simulink model "PIDusingOPAMP"  (R2015a)
settings: Solver=ode45  StartTime=0.0  StopTime=0.008  RelTol=1e-6
libraries: fl_lib x43, nesl_utility x2, powerlib x1
settings Model: Creator=my pc  LastModifiedBy=my pc

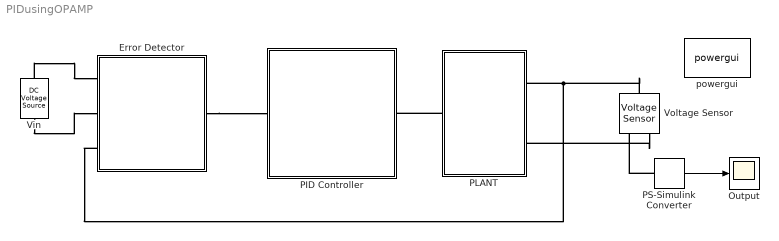
== system PIDusingOPAMP ==
  Error Detector : Subsystem
  Output : Scope
      settings: SaveName=PID
  PID Controller : Subsystem
  PLANT : Subsystem
  PS-Simulink Converter : nesl_utility/PS-Simulink Converter  PhysicalDomain=network_engine_domain  SubClassName=ps_output  LeftPortType=input  RightPortType=output  PseudoPeriodic=off  Frequencies=[]  Unit=1  AffineConversion=off
  Vin : fl_lib/Electrical/Electrical Sources/DC Voltage Source  v0=5 V
  Voltage Sensor : fl_lib/Electrical/Electrical Sensors/Voltage Sensor
  powergui : powerlib/powergui  Priority=1  SimulationMode=Continuous  SolverType=Tustin/Backward Euler (TBE)  SampleTime=50e-6  frequency=60  SPID=off  DisableSnubberDevices=off  DisableRonSwitches=off  DisableVfSwitches=off  SwTol=0  DisplayEquations=off  Interpol=off  methode=off  Ts=100  FunctionMessages=off  echomessages=off  HookPort=off  EnableUseOfTLC=off  x0status=blocks  frequencyindice=60  Pbase=100e6  ErrMax=1e-4  Iterations=50  UnitsV=kV  UnitsW=MW  buscounter=0  RestoreLinks=warning  ResistiveCurrentMeasurement=off  Frange=[0:2:500]  Ylog=off  Xlog=on  ShowGrid=off  save=off  variable=ZData  structure=0  ZoomFFT=off  StartTime=0.0  cycles=1  DisplayStyle=1  fundamental=60  FreqAxis=off  MaxFrequency=1000  frequencyindicesteady=1  RmsSteady=1  display=off
  wires:
  PS-Simulink Converter/1 -> Output/1
  connections:
  Voltage Sensor/LConn1 -- Error Detector/RConn3 -- PLANT/RConn1
  Voltage Sensor/RConn2 -- PLANT/RConn2
  Vin/LConn1 -- Error Detector/RConn1
  Vin/RConn1 -- Error Detector/RConn2
  Error Detector/LConn1 -- PID Controller/LConn1
  PS-Simulink Converter/LConn1 -- Voltage Sensor/RConn1
  PLANT/LConn1 -- PID Controller/RConn1

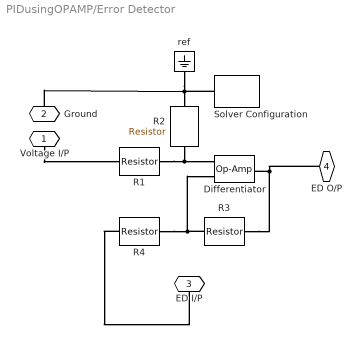
== system PIDusingOPAMP/Error Detector ==
  Differentiator : fl_lib/Electrical/Electrical Elements/Op-Amp  outI_specify=off  outI_priority=High  outI=0 A
  R{1..4} (4 alike) : fl_lib/Electrical/Electrical Elements/Resistor  R=4.7 kOhm  i_specify=off  i_priority=High  i=0 A  v_specify=off  v_priority=High  v=0 V
  Solver Configuration : nesl_utility/Solver Configuration  PhysicalDomain=network_engine_domain  SubClassName=solver  LeftPortType=input  RightPortType=generic  Accelerate=off  Tones=[]  Harmonics=[]  SimulateNoise=off  Profile=off  UseLocalSampling=off  EnableSwitchedLinearOptims=on  FrequencyDomain=off  UseCCode=off  RelTol=0.001  AbsTol=1e-06  MinStep=1e-09  ToWorkspace=off  RevertToSquareIcSolve=off  NumHomotopyIterations=100  DoDC=off  ResidualTolerance=1e-09  UseLocalSolver=off  LocalSolverChoice=NE_BACKWARD_EULER_ADVANCER  LocalSolverSampleTime=0.001  DoFixedCost=off  MaxNonlinIter=3  MaxModeIter=2  LinearAlgebra=Sparse  DelaysMemoryBudget=1024  AutomaticFiltering=on  FilteringTimeConstant=0.001
  ref : fl_lib/Electrical/Electrical Elements/Electrical Reference
  Voltage I/P : PMIOPort  Port=1  Side=Right
  Ground : PMIOPort  Port=2  Side=Right
  ED I/P : PMIOPort  Port=3  Side=Right
  ED O/P : PMIOPort  Port=4  Side=Left
  connections:
  R4/LConn1 -- ED I/P/RConn1
  Voltage I/P/RConn1 -- R1/LConn1
  R1/RConn1 -- R2/LConn1 -- Differentiator/LConn1
  ref/LConn1 -- Ground/RConn1 -- Solver Configuration/RConn1 -- R2/RConn1
  R4/RConn1 -- R3/RConn1 -- Differentiator/LConn2
  R3/LConn1 -- ED O/P/RConn1 -- Differentiator/RConn1

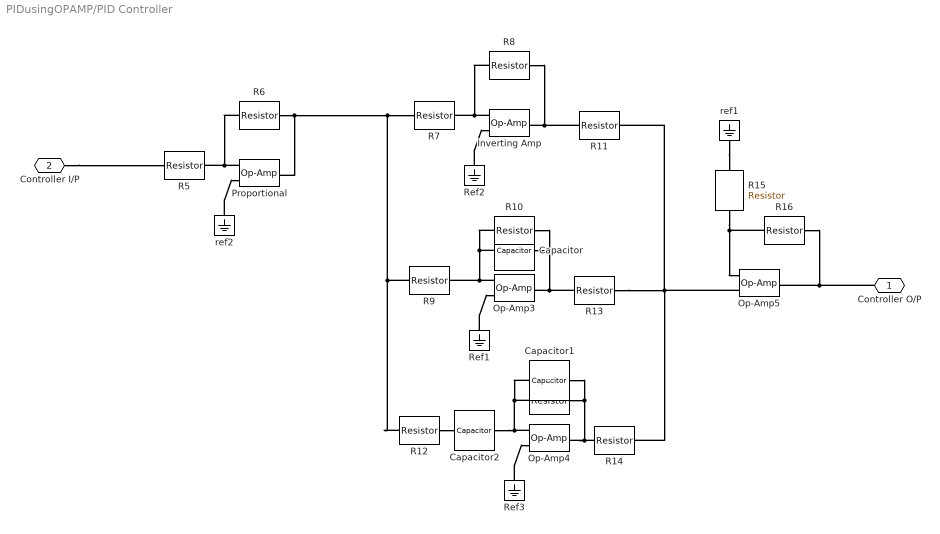
== system PIDusingOPAMP/PID Controller ==
  . : fl_lib/Electrical/Electrical Elements/Resistor  R=5.93 kOhm  i_specify=off  i_priority=High  i=0 A  v_specify=off  v_priority=High  v=0 V
  Capacitor : fl_lib/Electrical/Electrical Elements/Capacitor  c=1 uF  r=1e-6 Ohm  g=0 1/Ohm  i_specify=off  i_priority=High  i=0 A  v_specify=off  v_priority=High  v=0 V  vc_specify=off  vc_priority=High  vc=0 V
  Capacitor1 : fl_lib/Electrical/Electrical Elements/Capacitor  c=1 nF  r=1e-6 Ohm  g=0 1/Ohm  i_specify=off  i_priority=High  i=0 A  v_specify=off  v_priority=High  v=0 V  vc_specify=off  vc_priority=High  vc=0 V
  Capacitor2 : fl_lib/Electrical/Electrical Elements/Capacitor  c=0.3 uF  r=1e-6 Ohm  g=0 1/Ohm  i_specify=off  i_priority=High  i=0 A  v_specify=off  v_priority=High  v=0 V  vc_specify=off  vc_priority=High  vc=0 V
  Inverting Amp : fl_lib/Electrical/Electrical Elements/Op-Amp  outI_specify=off  outI_priority=High  outI=0 A
  Op-Amp3 : fl_lib/Electrical/Electrical Elements/Op-Amp  outI_specify=off  outI_priority=High  outI=0 A
  Op-Amp4 : fl_lib/Electrical/Electrical Elements/Op-Amp  outI_specify=off  outI_priority=High  outI=0 A
  Op-Amp5 : fl_lib/Electrical/Electrical Elements/Op-Amp  outI_specify=off  outI_priority=High  outI=0 A
  Proportional : fl_lib/Electrical/Electrical Elements/Op-Amp  outI_specify=off  outI_priority=High  outI=0 A
  R10 : fl_lib/Electrical/Electrical Elements/Resistor  R=2.37 kOhm  i_specify=off  i_priority=High  i=0 A  v_specify=off  v_priority=High  v=0 V
  R{5,7..8,11,13..15} (7 alike) : fl_lib/Electrical/Electrical Elements/Resistor  R=1 kOhm  i_specify=off  i_priority=High  i=0 A  v_specify=off  v_priority=High  v=0 V
  R12 : fl_lib/Electrical/Electrical Elements/Resistor  R=59 Ohm  i_specify=off  i_priority=High  i=0 A  v_specify=off  v_priority=High  v=0 V
  R16 : fl_lib/Electrical/Electrical Elements/Resistor  R=2 kOhm  i_specify=off  i_priority=High  i=0 A  v_specify=off  v_priority=High  v=0 V
  R6 : fl_lib/Electrical/Electrical Elements/Resistor  R=8.1 kOhm  i_specify=off  i_priority=High  i=0 A  v_specify=off  v_priority=High  v=0 V
  R9 : fl_lib/Electrical/Electrical Elements/Resistor  R=23.7 kOhm  i_specify=off  i_priority=High  i=0 A  v_specify=off  v_priority=High  v=0 V
  Ref1 : fl_lib/Electrical/Electrical Elements/Electrical Reference
  Ref2 : fl_lib/Electrical/Electrical Elements/Electrical Reference
  Ref3 : fl_lib/Electrical/Electrical Elements/Electrical Reference
  ref1 : fl_lib/Electrical/Electrical Elements/Electrical Reference
  ref2 : fl_lib/Electrical/Electrical Elements/Electrical Reference
  Controller O/P : PMIOPort  Port=1  Side=Right
  Controller I/P : PMIOPort  Port=2  Side=Left
  connections:
  R9/RConn1 -- Op-Amp3/LConn2 -- Capacitor/RConn1 -- R10/RConn1
  Op-Amp3/RConn1 -- R13/LConn1 -- R10/LConn1 -- Capacitor/LConn1
  R13/RConn1 -- R11/RConn1 -- R14/RConn1 -- Op-Amp5/LConn1
  Capacitor1/LConn1 -- R14/LConn1 -- Op-Amp4/RConn1 -- ./LConn1
  Capacitor1/RConn1 -- ./RConn1 -- Op-Amp4/LConn2 -- Capacitor2/RConn1
  Proportional/RConn1 -- R7/LConn1 -- R12/LConn1 -- R9/LConn1 -- R6/LConn1
  Ref1/LConn1 -- Op-Amp3/LConn1
  R12/RConn1 -- Capacitor2/LConn1
  Ref3/LConn1 -- Op-Amp4/LConn1
  Inverting Amp/RConn1 -- R8/LConn1 -- R11/LConn1
  R7/RConn1 -- Inverting Amp/LConn2 -- R8/RConn1
  Ref2/LConn1 -- Inverting Amp/LConn1
  R5/RConn1 -- Proportional/LConn2 -- R6/RConn1
  ref2/LConn1 -- Proportional/LConn1
  Controller I/P/RConn1 -- R5/LConn1
  R15/RConn1 -- R16/RConn1 -- Op-Amp5/LConn2
  Op-Amp5/RConn1 -- Controller O/P/RConn1 -- R16/LConn1
  ref1/LConn1 -- R15/LConn1

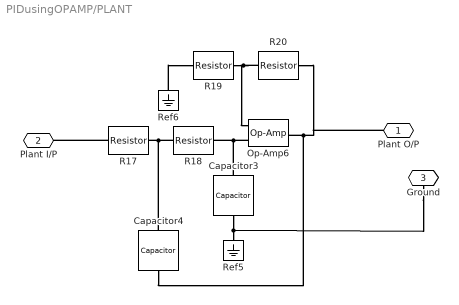
== system PIDusingOPAMP/PLANT ==
  Capacitor3 : fl_lib/Electrical/Electrical Elements/Capacitor  c=1 uF  r=1e-6 Ohm  g=0 1/Ohm  i_specify=off  i_priority=High  i=0 A  v_specify=off  v_priority=High  v=0 V  vc_specify=off  vc_priority=High  vc=0 V
  Capacitor4 : fl_lib/Electrical/Electrical Elements/Capacitor  c=1 uF  r=1e-6 Ohm  g=0 1/Ohm  i_specify=off  i_priority=High  i=0 A  v_specify=off  v_priority=High  v=0 V  vc_specify=off  vc_priority=High  vc=0 V
  Op-Amp6 : fl_lib/Electrical/Electrical Elements/Op-Amp  outI_specify=off  outI_priority=High  outI=0 A
  R17 : fl_lib/Electrical/Electrical Elements/Resistor  R=4.7 kOhm  i_specify=off  i_priority=High  i=0 A  v_specify=off  v_priority=High  v=0 V
  R18 : fl_lib/Electrical/Electrical Elements/Resistor  R=4.7 kOhm  i_specify=off  i_priority=High  i=0 A  v_specify=off  v_priority=High  v=0 V
  R19 : fl_lib/Electrical/Electrical Elements/Resistor  R=4.7 kOhm  i_specify=off  i_priority=High  i=0 A  v_specify=off  v_priority=High  v=0 V
  R20 : fl_lib/Electrical/Electrical Elements/Resistor  R=9.3 kOhm  i_specify=off  i_priority=High  i=0 A  v_specify=off  v_priority=High  v=0 V
  Ref5 : fl_lib/Electrical/Electrical Elements/Electrical Reference
  Ref6 : fl_lib/Electrical/Electrical Elements/Electrical Reference
  Plant O/P : PMIOPort  Port=1  Side=Right
  Plant I/P : PMIOPort  Port=2  Side=Left
  Ground : PMIOPort  Port=3  Side=Right
  connections:
  R18/LConn1 -- R17/RConn1 -- Capacitor4/LConn1
  Op-Amp6/LConn1 -- Capacitor3/LConn1 -- R18/RConn1
  Ref6/LConn1 -- R19/LConn1
  Capacitor3/RConn1 -- Ground/RConn1 -- Ref5/LConn1
  R19/RConn1 -- R20/RConn1 -- Op-Amp6/LConn2
  Capacitor4/RConn1 -- Plant O/P/RConn1 -- R20/LConn1 -- Op-Amp6/RConn1
  R17/LConn1 -- Plant I/P/RConn1
